simulink model "Boat_Simulation_V1"  (R2015a)
settings: Solver=ode45  StartTime=0.0  StopTime=50  RelTol=1e-3
values from neighbouring files (symbols this model uses):
  d_cg = [0 0 0]    [boatVars.m]
  d_motors = w_boat-0.02    (= 0.06)    [boatVars.m]
  Izz_boat = 1    [boatVars.m]
  k_drag_para = 1    [boatVars.m]
  k_drag_perp = 1    [boatVars.m]
  k_drag_rot = 0.4    [boatVars.m]
  m_boat = 0.120    (= 0.12)    [boatVars.m]
  theta0_boat = 0.*pi/180    (= 0)    [boatVars.m]
  theta_dot0_boat = 0    [boatVars.m]
  use_imu_model = 0    [boatVars.m]
  v0_boat = [0 0]    [boatVars.m]
  x0_boat = waypoints_load(1,:)    [boatVars.m]
  xd = part_pos_2(ii-1,1)    [Baseline_on_Sim.m]    (also in TrackExample.m; TrackExample_revised.m; boatVars.m = 1.5)
  xs = linspace(0,lambda_field,nx)    [boatVars.m]    (also in efficientPath_trials.m = 0:xStep:2*yy; grid_define.m = xmin:step:xmax)
  yd = part_pos_2(ii-1,2)    [Baseline_on_Sim.m]    (also in TrackExample.m; TrackExample_revised.m; boatVars.m = 0.5)
  ys = linspace(0,b_field,ny)    [boatVars.m]    (also in efficientPath_trials.m = 0:yStep:yy; grid_define.m = ymin:step:ymax)
undefined symbols (not defined in the file): b_motor, J_motor, kphi_motor, L_motor, R_motor
libraries: simulink x2, aerolibnav x1
settings Model: Creator=Jack  LastModifiedBy=Jack

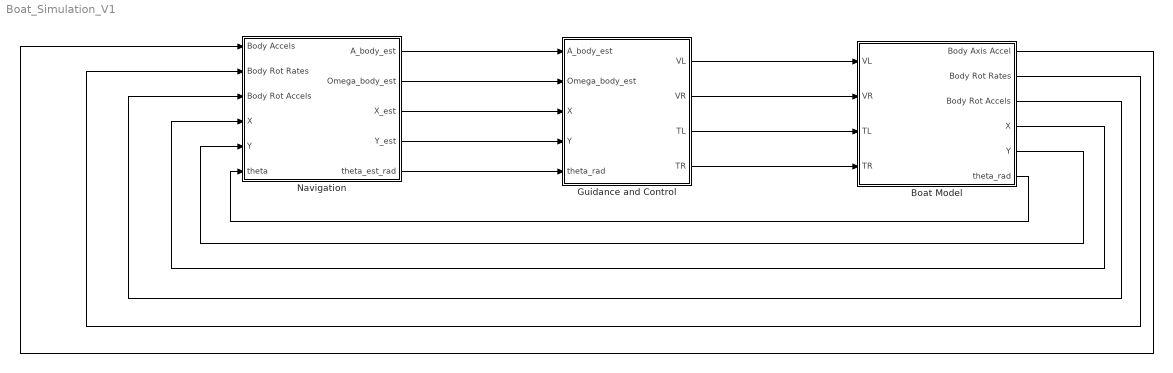
== system Boat_Simulation_V1 ==
  Boat Model : Subsystem
  Guidance and Control : Subsystem
  Navigation : Subsystem
  wires:
  Boat Model/1(Body Axis Accel) -> Navigation/1(Body Accels)
  Boat Model/2(Body Rot Rates) -> Navigation/2(Body Rot Rates)
  Boat Model/3(Body Rot Accels) -> Navigation/3(Body Rot Accels)
  Navigation/1(A_body_est) -> Guidance and Control/1(A_body_est)
  Navigation/2(Omega_body_est) -> Guidance and Control/2(Omega_body_est)
  Guidance and Control/1(VL) -> Boat Model/1(VL)
  Guidance and Control/2(VR) -> Boat Model/2(VR)
  Guidance and Control/3(TL) -> Boat Model/3(TL)
  Guidance and Control/4(TR) -> Boat Model/4(TR)
  Boat Model/4(X) -> Navigation/4(X)
  Boat Model/5(Y) -> Navigation/5(Y)
  Navigation/3(X_est) -> Guidance and Control/3(X)
  Navigation/4(Y_est) -> Guidance and Control/4(Y)
  Navigation/5(theta_est_rad) -> Guidance and Control/5(theta_rad)
  Boat Model/6(theta_rad) -> Navigation/6(theta)

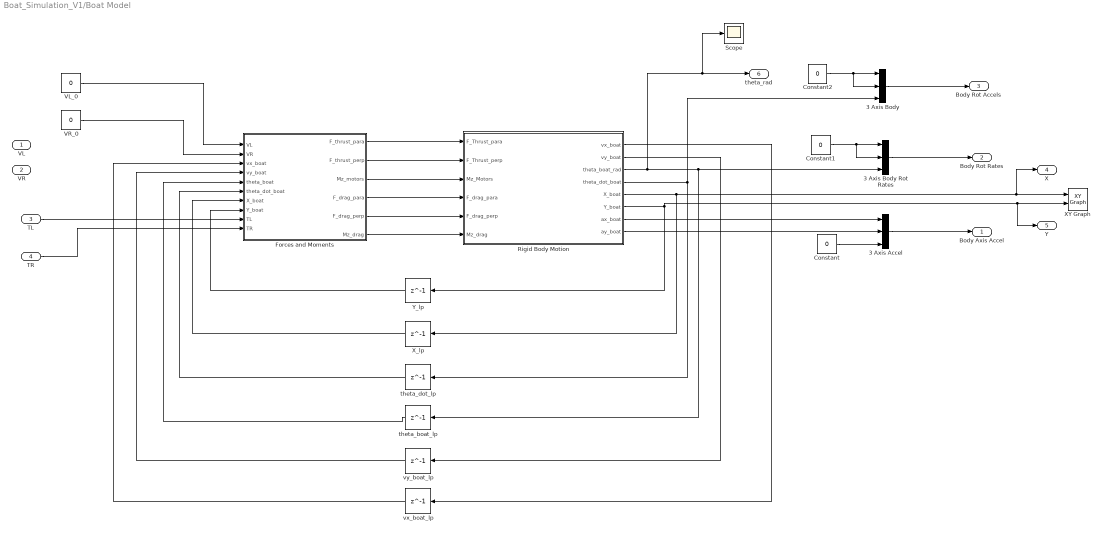
== system Boat_Simulation_V1/Boat Model ==
  VL : Inport
  VR : Inport  Port=2
  TL : Inport  Port=3
  TR : Inport  Port=4
  3 Axis Accel : Concatenate  NumInputs=3
  3 Axis Body : Concatenate  NumInputs=3
  3 Axis Body Rot Rates : Concatenate  NumInputs=3
  Constant : Constant  Value=0
  Constant1 : Constant  Value=0
  Constant2 : Constant  Value=0
  Forces and Moments : Subsystem
  Rigid Body Motion : Subsystem
  Scope : Scope
      settings: SaveName=ScopeData5
  VL_0 : Constant  Value=0
  VR_0 : Constant  Value=0
  XY Graph : simulink/Sinks/XY Graph  xmin=0  xmax=2  ymin=0  ymax=1  st=0.01
  X_lp : Delay  DelayLength=1  InitialCondition=x0_boat(1)  SampleTime=0.01
  Y_lp : Delay  DelayLength=1  InitialCondition=x0_boat(2)  SampleTime=0.01
  theta_boat_lp : Delay  DelayLength=1  InitialCondition=theta0_boat  SampleTime=0.01
  theta_dot_lp : Delay  DelayLength=1  InitialCondition=theta_dot0_boat  SampleTime=0.01
  vx_boat_lp : Delay  DelayLength=1  InitialCondition=v0_boat(1)  SampleTime=0.01
  vy_boat_lp : Delay  DelayLength=1  InitialCondition=v0_boat(2)  SampleTime=0.01
  Body Axis Accel : Outport
  Body Rot Rates : Outport  Port=2
  Body Rot Accels : Outport  Port=3
  X : Outport  Port=4
  Y : Outport  Port=5
  theta_rad : Outport  Port=6
  wires:
  Forces and Moments/3(Mz_motors) -> Rigid Body Motion/3(Mz_Motors)
  Forces and Moments/2(F_thrust_perp) -> Rigid Body Motion/2(F_Thrust_perp)
  Forces and Moments/1(F_thrust_para) -> Rigid Body Motion/1(F_Thrust_para)
  Forces and Moments/4(F_drag_para) -> Rigid Body Motion/4(F_drag_para)
  Forces and Moments/5(F_drag_perp) -> Rigid Body Motion/5(F_drag_perp)
  Forces and Moments/6(Mz_drag) -> Rigid Body Motion/6(Mz_drag)
  Rigid Body Motion/1(vx_boat) -> vx_boat_lp/1
  Rigid Body Motion/2(vy_boat) -> vy_boat_lp/1
  VL_0/1 -> Forces and Moments/1(VL)
  VR_0/1 -> Forces and Moments/2(VR)
  Rigid Body Motion/5(X_boat) -> X_lp/1, X/1, XY Graph/1
  Rigid Body Motion/6(Y_boat) -> Y_lp/1, Y/1, XY Graph/2
  vx_boat_lp/1 -> Forces and Moments/3(vx_boat)
  vy_boat_lp/1 -> Forces and Moments/4(vy_boat)
  theta_boat_lp/1 -> Forces and Moments/5(theta_boat)
  theta_dot_lp/1 -> Forces and Moments/6(theta_dot_boat)
  X_lp/1 -> Forces and Moments/7(X_boat)
  Y_lp/1 -> Forces and Moments/8(Y_boat)
  Rigid Body Motion/7(ax_boat) -> 3 Axis Accel/1
  3 Axis Accel/1 -> Body Axis Accel/1
  Rigid Body Motion/8(ay_boat) -> 3 Axis Accel/2
  Constant/1 -> 3 Axis Accel/3
  3 Axis Body Rot Rates/1 -> Body Rot Rates/1
  Constant1/1 -> 3 Axis Body Rot Rates/2, 3 Axis Body Rot Rates/1
  Rigid Body Motion/4(theta_dot_boat) -> theta_dot_lp/1, 3 Axis Body/3
  3 Axis Body/1 -> Body Rot Accels/1
  Constant2/1 -> 3 Axis Body/2, 3 Axis Body/1
  TL/1 -> Forces and Moments/9(TL)
  TR/1 -> Forces and Moments/10(TR)
  Rigid Body Motion/3(theta_boat_rad) -> Scope/1, theta_rad/1, 3 Axis Body Rot Rates/3, theta_boat_lp/1

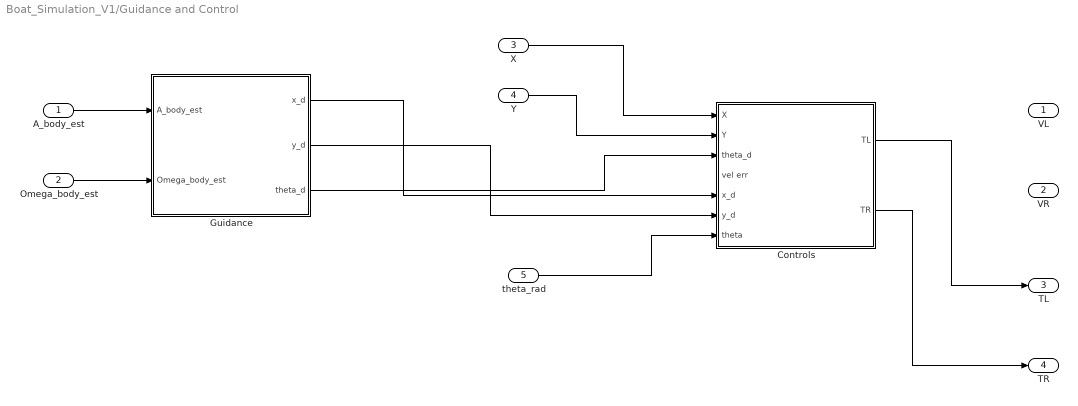
== system Boat_Simulation_V1/Guidance and Control ==
  A_body_est : Inport
  Omega_body_est : Inport  Port=2
  X : Inport  Port=3
  Y : Inport  Port=4
  theta_rad : Inport  Port=5
  Controls : Subsystem
  Guidance : Subsystem
  VL : Outport
  VR : Outport  Port=2
  TL : Outport  Port=3
  TR : Outport  Port=4
  wires:
  Omega_body_est/1 -> Guidance/2("Omega_body_est ")
  A_body_est/1 -> Guidance/1(A_body_est)
  X/1 -> Controls/1(X)
  Y/1 -> Controls/2(Y)
  Guidance/1(x_d) -> Controls/5(x_d)
  Guidance/2(y_d) -> Controls/6(y_d)
  Guidance/3(theta_d) -> Controls/3(theta_d)
  Controls/1(TL) -> TL/1
  Controls/2(TR) -> TR/1
  theta_rad/1 -> Controls/7(theta)

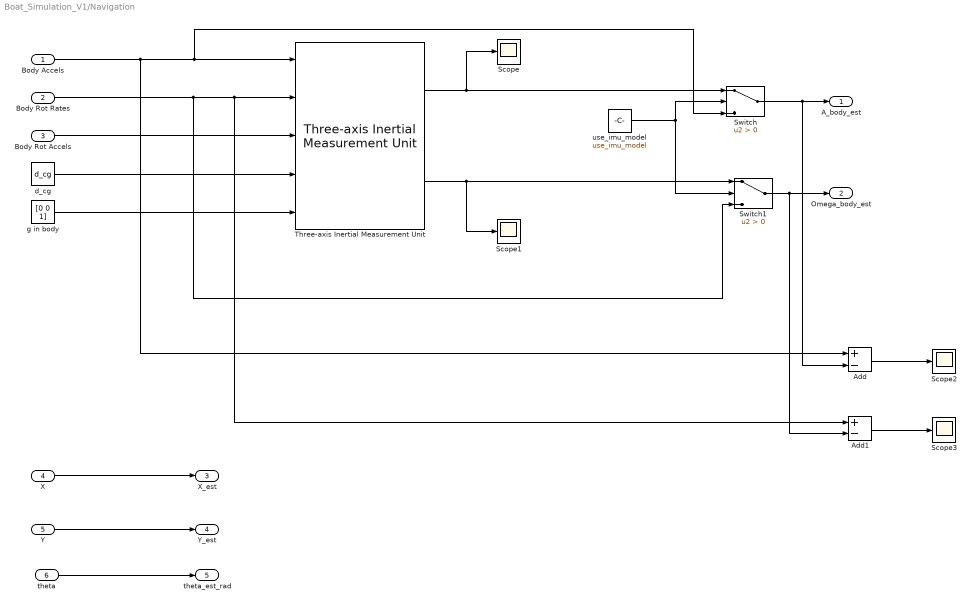
== system Boat_Simulation_V1/Navigation ==
  Body Accels : Inport
  Body Rot Rates : Inport  Port=2
  Body Rot Accels : Inport  Port=3
  X : Inport  Port=4
  Y : Inport  Port=5
  theta : Inport  Port=6
  Add : Sum  Inputs=+-
  Add1 : Sum  Inputs=+-
  Scope{,1..3} (4 alike) : Scope
      Scope settings: ShowLegends=on
      Scope1 settings: ShowLegends=on
      Scope2 settings: SaveName=ScopeData2
      Scope3 settings: SaveName=ScopeData3
  Switch : Switch  Criteria=u2 > Threshold
  Switch1 : Switch  Criteria=u2 > Threshold
  Three-axis Inertial Measurement Unit : aerolibnav/Three-axis Inertial Measurement Unit  units=Metric (MKS)  imu=[0 0 0]  dtype_a=on  w_a=190  z_a=0.707  a_sf_cc=[1 0 0; 0 1 0; 0 0 1]  a_bias=[0 0 0]  a_sat="[-inf  -inf  -inf  inf inf inf]"  dtype_g=on  w_g=190  z_g=0.707  g_sf_cc=[1 0 0; 0 1 0; 0 0 1]  g_bias=[0 0 0]  g_sens=[0 0 0]  g_sat="[-inf  -inf  -inf  inf inf inf]"  i_rand=on  i_seeds=[23093 23094 23095 23096 23097 23098]  i_pow=[0.001 0.001 0.001 0.0001 0.0001 0.0001]  i_Ts=0
  d_cg : Constant  Value=d_cg
  "g in body " : Constant  Value=[0 0 1]
  use_imu_model : Constant  Value=use_imu_model
  A_body_est : Outport
  Omega_body_est : Outport  Port=2
  X_est : Outport  Port=3
  Y_est : Outport  Port=4
  theta_est_rad : Outport  Port=5
  wires:
  Body Accels/1 -> Add/1, Switch/3, Three-axis Inertial Measurement Unit/1
  Body Rot Rates/1 -> Switch1/3, Add1/1, Three-axis Inertial Measurement Unit/2
  Body Rot Accels/1 -> Three-axis Inertial Measurement Unit/3
  "g in body "/1 -> Three-axis Inertial Measurement Unit/5
  d_cg/1 -> Three-axis Inertial Measurement Unit/4
  Three-axis Inertial Measurement Unit/1 -> Switch/1, Scope/1
  Three-axis Inertial Measurement Unit/2 -> Switch1/1, Scope1/1
  Switch1/1 -> Add1/2, Omega_body_est/1
  Switch/1 -> Add/2, A_body_est/1
  use_imu_model/1 -> Switch1/2, Switch/2
  Add/1 -> Scope2/1
  Add1/1 -> Scope3/1
  X/1 -> X_est/1
  Y/1 -> Y_est/1
  theta/1 -> theta_est_rad/1

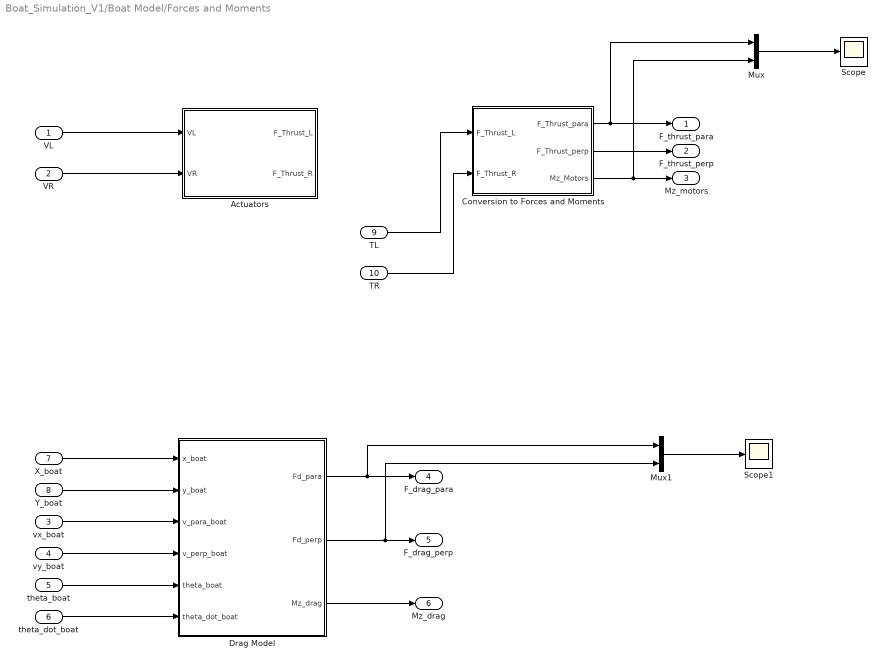
== system Boat_Simulation_V1/Boat Model/Forces and Moments ==
  VL : Inport
  VR : Inport  Port=2
  vx_boat : Inport  Port=3
  vy_boat : Inport  Port=4
  theta_boat : Inport  Port=5
  theta_dot_boat : Inport  Port=6
  X_boat : Inport  Port=7
  Y_boat : Inport  Port=8
  TL : Inport  Port=9
  TR : Inport  Port=10
  Actuators : Subsystem
  Conversion to Forces and Moments : Subsystem
  Drag Model : Subsystem
  Mux : Mux  Inputs=2
  Mux1 : Mux  Inputs=2
  Scope : Scope
      settings: SaveName=ScopeData4
  Scope1 : Scope
      settings: SaveName=ScopeData6
  F_thrust_para : Outport
  F_thrust_perp : Outport  Port=2
  Mz_motors : Outport  Port=3
  F_drag_para : Outport  Port=4
  F_drag_perp : Outport  Port=5
  Mz_drag : Outport  Port=6
  wires:
  VR/1 -> Actuators/2(VR)
  VL/1 -> Actuators/1(VL)
  X_boat/1 -> Drag Model/1(x_boat)
  Y_boat/1 -> Drag Model/2(y_boat)
  vx_boat/1 -> Drag Model/3(v_para_boat)
  vy_boat/1 -> Drag Model/4(v_perp_boat)
  theta_boat/1 -> Drag Model/5(theta_boat)
  Drag Model/3(Mz_drag) -> Mz_drag/1
  Conversion to Forces and Moments/1(F_Thrust_para) -> Mux/1, F_thrust_para/1
  Conversion to Forces and Moments/2(F_Thrust_perp) -> F_thrust_perp/1
  Conversion to Forces and Moments/3(Mz_Motors) -> Mux/2, Mz_motors/1
  theta_dot_boat/1 -> Drag Model/6(theta_dot_boat)
  TL/1 -> Conversion to Forces and Moments/1(F_Thrust_L)
  TR/1 -> Conversion to Forces and Moments/2(F_Thrust_R)
  Mux/1 -> Scope/1
  Drag Model/1(Fd_para) -> Mux1/1, F_drag_para/1
  Drag Model/2(Fd_perp) -> Mux1/2, F_drag_perp/1
  Mux1/1 -> Scope1/1

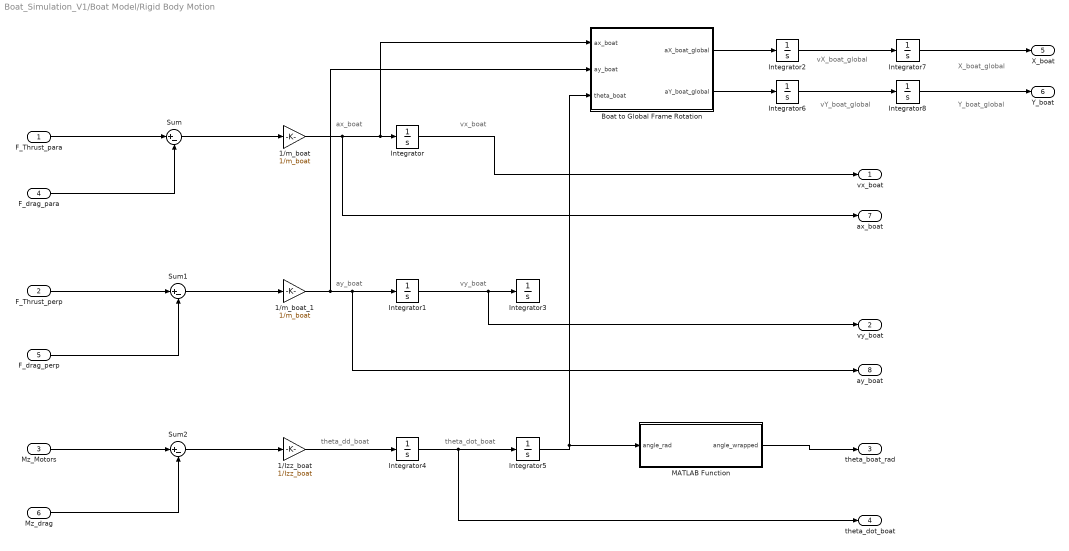
== system Boat_Simulation_V1/Boat Model/Rigid Body Motion ==
  note: Y_boat_global
  note: X_boat_global
  note: vX_boat_global
  note: ax_boat
  note: ay_boat
  note: vx_boat
  note: vy_boat
  note: theta_dd_boat
  note: theta_dot_boat
  note: vY_boat_global
  F_Thrust_para : Inport
  F_Thrust_perp : Inport  Port=2
  Mz_Motors : Inport  Port=3
  F_drag_para : Inport  Port=4
  F_drag_perp : Inport  Port=5
  Mz_drag : Inport  Port=6
  " Boat to Global Frame Rotation" : Subsystem
  1/Izz_boat : Gain  Gain=1/Izz_boat
  1/m_boat : Gain  Gain=1/m_boat
  1/m_boat_1 : Gain  Gain=1/m_boat
  Integrator : Integrator
  Integrator1 : Integrator
  Integrator2 : Integrator  InitialCondition=v0_boat(1)
  Integrator3 : Integrator
  Integrator4 : Integrator  InitialCondition=theta_dot0_boat
  Integrator5 : Integrator  InitialCondition=theta0_boat
  Integrator6 : Integrator  InitialCondition=v0_boat(2)
  Integrator7 : Integrator  InitialCondition=x0_boat(1)  LimitOutput=on  UpperSaturationLimit=2  LowerSaturationLimit=0
  Integrator8 : Integrator  InitialCondition=x0_boat(2)  LimitOutput=on  UpperSaturationLimit=1  LowerSaturationLimit=0
  MATLAB Function : MATLAB Function  TreatAsAtomicUnit=on
  Sum : Sum  Inputs=|+-
  Sum1 : Sum  Inputs=|+-
  Sum2 : Sum  Inputs=|+-
  vx_boat : Outport
  vy_boat : Outport  Port=2
  theta_boat_rad : Outport  Port=3
  theta_dot_boat : Outport  Port=4
  X_boat : Outport  Port=5
  Y_boat : Outport  Port=6
  ax_boat : Outport  Port=7
  ay_boat : Outport  Port=8
  wires:
  F_Thrust_para/1 -> Sum/1
  F_drag_para/1 -> Sum/2
  Sum/1 -> 1/m_boat/1
  Sum1/1 -> 1/m_boat_1/1
  F_Thrust_perp/1 -> Sum1/1
  F_drag_perp/1 -> Sum1/2
  1/m_boat/1 -> ax_boat/1, " Boat to Global Frame Rotation"/1(ax_boat), Integrator/1
  Integrator/1 -> vx_boat/1
  Integrator1/1 -> vy_boat/1, Integrator3/1
  Mz_Motors/1 -> Sum2/1
  Mz_drag/1 -> Sum2/2
  Sum2/1 -> 1/Izz_boat/1
  1/Izz_boat/1 -> Integrator4/1
  Integrator4/1 -> theta_dot_boat/1, Integrator5/1
  Integrator5/1 -> " Boat to Global Frame Rotation"/3(theta_boat), MATLAB Function/1(angle_rad)
  " Boat to Global Frame Rotation"/1(aX_boat_global) -> Integrator2/1
  " Boat to Global Frame Rotation"/2(aY_boat_global) -> Integrator6/1
  Integrator2/1 -> Integrator7/1
  Integrator6/1 -> Integrator8/1
  Integrator7/1 -> X_boat/1
  Integrator8/1 -> Y_boat/1
  1/m_boat_1/1 -> " Boat to Global Frame Rotation"/2(ay_boat), ay_boat/1, Integrator1/1
  MATLAB Function/1(angle_wrapped) -> theta_boat_rad/1

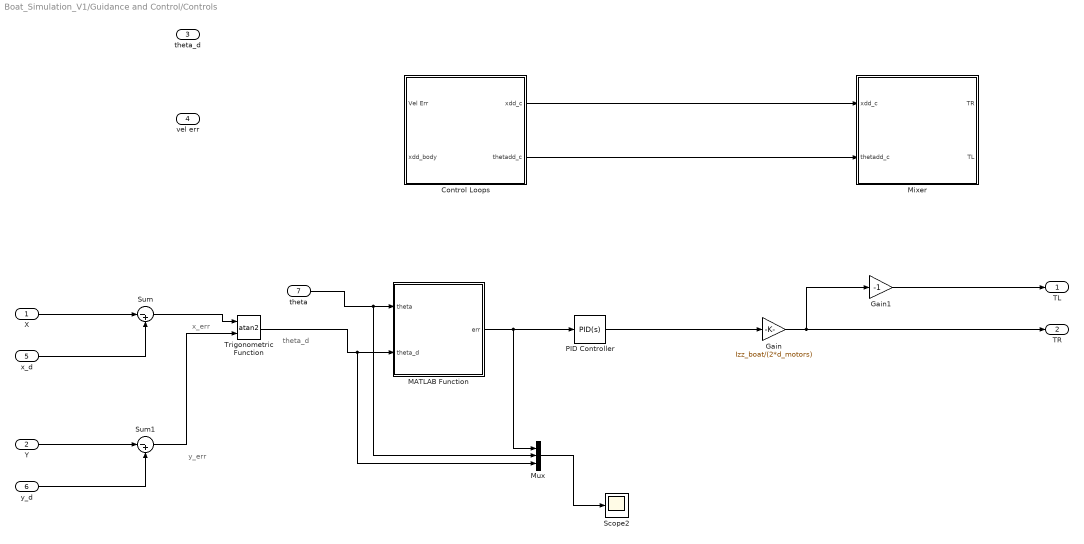
== system Boat_Simulation_V1/Guidance and Control/Controls ==
  note: theta_d
  note: y_err
  note: x_err
  X : Inport
  Y : Inport  Port=2
  theta_d : Inport  Port=3
  vel err : Inport  Port=4
  x_d : Inport  Port=5
  y_d : Inport  Port=6
  theta : Inport  Port=7
  Control Loops : Subsystem
  Gain : Gain  Gain=Izz_boat/(2*d_motors)
  Gain1 : Gain  Gain=-1
  MATLAB Function : MATLAB Function  TreatAsAtomicUnit=on
  Mixer : Subsystem
  Mux : Mux  Inputs=3
  PID Controller : simulink/Continuous/PID Controller  Controller=PID  TimeDomain=Continuous-time  SampleTime=-1  IntegratorMethod=Forward Euler  FilterMethod=Forward Euler  Form=Parallel  UseFilter=on  ControllerParametersSource=internal  P=0.3  I=0.1  D=0  N=100  InitialConditionSource=internal  InitialConditionForIntegrator=0  InitialConditionForFilter=0  ExternalReset=none  LimitOutput=off  UpperSaturationLimit=inf  LowerSaturationLimit=-inf  LinearizeAsGain=on  AntiWindupMode=none  Kb=1  TrackingMode=off  Kt=1  PParamMin=[]  PParamMax=[]  IParamMin=[]  IParamMax=[]  DParamMin=[]  DParamMax=[]  NParamMin=[]  NParamMax=[]  KbParamMin=[]  KbParamMax=[]  KtParamMin=[]  KtParamMax=[]  POutMin=[]  POutMax=[]  IOutMin=[]  IOutMax=[]  DOutMin=[]  DOutMax=[]  NOutMin=[]  NOutMax=[]  KbOutMin=[]  KbOutMax=[]  KtOutMin=[]  KtOutMax=[]  IntegratorOutMin=[]  IntegratorOutMax=[]  FilterOutMin=[]  FilterOutMax=[]  SumOutMin=[]  SumOutMax=[]  SumI1OutMin=[]  SumI1OutMax=[]  SumI2OutMin=[]  SumI2OutMax=[]  SumI3OutMin=[]  SumI3OutMax=[]  SumDOutMin=[]  SumDOutMax=[]  SaturationOutMin=[]  SaturationOutMax=[]  IntegratorContinuousStateAttributes=''  IntegratorStateMustResolveToSignalObject=off  IntegratorRTWStateStorageClass=Auto  FilterContinuousStateAttributes=''  FilterStateMustResolveToSignalObject=off  FilterRTWStateStorageClass=Auto  DifferentiatorICPrevScaledInput=0  DifferentiatorOutMin=[]  DifferentiatorOutMax=[]
  Scope2 : Scope
      settings: ShowLegends=on  SaveName=ScopeData9
  Sum : Sum  Inputs=|-+
  Sum1 : Sum  Inputs=|-+
  Trigonometric Function : Trigonometry  Operator=atan2
  TL : Outport
  TR : Outport  Port=2
  wires:
  Control Loops/1(xdd_c) -> Mixer/1(xdd_c)
  Control Loops/2(thetadd_c) -> Mixer/2(thetadd_c)
  X/1 -> Sum/1
  x_d/1 -> Sum/2
  Y/1 -> Sum1/1
  y_d/1 -> Sum1/2
  PID Controller/1 -> Gain/1
  Gain/1 -> TR/1, Gain1/1
  theta/1 -> Mux/2, MATLAB Function/1(theta)
  Sum/1 -> Trigonometric Function/1
  Sum1/1 -> Trigonometric Function/2
  Gain1/1 -> TL/1
  Mux/1 -> Scope2/1
  MATLAB Function/1(err) -> Mux/1, PID Controller/1
  Trigonometric Function/1 -> Mux/3, MATLAB Function/2(theta_d)

== system Boat_Simulation_V1/Guidance and Control/Guidance ==
  A_body_est : Inport
  "Omega_body_est " : Inport  Port=2
  Sine Wave : Sin  Amplitude=pi  Frequency=2*pi/50  SampleTime=0
  xd : Constant  Value=xd
  yd : Constant  Value=yd
  x_d : Outport
  y_d : Outport  Port=2
  theta_d : Outport  Port=3
  wires:
  xd/1 -> x_d/1
  yd/1 -> y_d/1
  Sine Wave/1 -> theta_d/1

== system Boat_Simulation_V1/Boat Model/Forces and Moments/Actuators ==
  note: Left Motor
  note: Right Motor
  VL : Inport
  VR : Inport  Port=2
  DC motor : Subsystem  mask(DC Motor){L=L_motor, Kphi=kphi_motor, J=J_motor, b=b_motor, R=R_motor}
      mask help:
      | Takes the DC voltage as input, and outputs angular velocity (w) and current (i)
      | L => windings inductance		Kphi => emf constant
      | J => loads moment of inertial		b => viscous friction
      | R => windings resistance
      mask Display:
      | port_label('input', 1, 'V')
      | port_label('output', 2, 'i')
      | port_label('output', 1, 'w')
      | disp('DC Motor')
  DC motor1 : Subsystem  mask(DC Motor){L=L_motor, Kphi=kphi_motor, J=J_motor, b=b_motor, R=R_motor}
      mask help:
      | Takes the DC voltage as input, and outputs angular velocity (w) and current (i)
      | L => windings inductance		Kphi => emf constant
      | J => loads moment of inertial		b => viscous friction
      | R => windings resistance
      mask Display:
      | port_label('input', 1, 'V')
      | port_label('output', 2, 'i')
      | port_label('output', 1, 'w')
      | disp('DC Motor')
  Prop Angular Velocity to Thrust : Lookup_n-D  NumberOfTableDimensions=1  BreakpointsForDimension1=[-5:5]  Table=tanh([-5:5])  InternalRulePriority=Speed  RndMeth=Simplest  InputSameDT=on
  Prop Angular Velocity to Thrust1 : Lookup_n-D  NumberOfTableDimensions=1  BreakpointsForDimension1=[-5:5]  Table=tanh([-5:5])  InternalRulePriority=Speed  RndMeth=Simplest  InputSameDT=on
  F_Thrust_L : Outport
  F_Thrust_R : Outport  Port=2
  wires:
  DC motor/1(w) -> Prop Angular Velocity to Thrust/1
  DC motor1/1(w) -> Prop Angular Velocity to Thrust1/1
  VL/1 -> DC motor/1(V)
  VR/1 -> DC motor1/1(V)
  Prop Angular Velocity to Thrust/1 -> F_Thrust_L/1
  Prop Angular Velocity to Thrust1/1 -> F_Thrust_R/1

== system Boat_Simulation_V1/Boat Model/Forces and Moments/Conversion to Forces and Moments ==
  F_Thrust_L : Inport
  F_Thrust_R : Inport  Port=2
  Constant : Constant  Value=0
  Divide : Product  Inputs=*/
  Sum : Sum  Inputs=|++
  Sum1 : Sum  Inputs=+-|
  d_motors/2 : Constant  Value=d_motors/2
  F_Thrust_para : Outport
  F_Thrust_perp : Outport  Port=2
  Mz_Motors : Outport  Port=3
  wires:
  F_Thrust_L/1 -> Sum1/1, Sum/1
  F_Thrust_R/1 -> Sum1/2, Sum/2
  Sum/1 -> F_Thrust_para/1
  Constant/1 -> F_Thrust_perp/1
  Sum1/1 -> Divide/1
  d_motors/2/1 -> Divide/2
  Divide/1 -> Mz_Motors/1

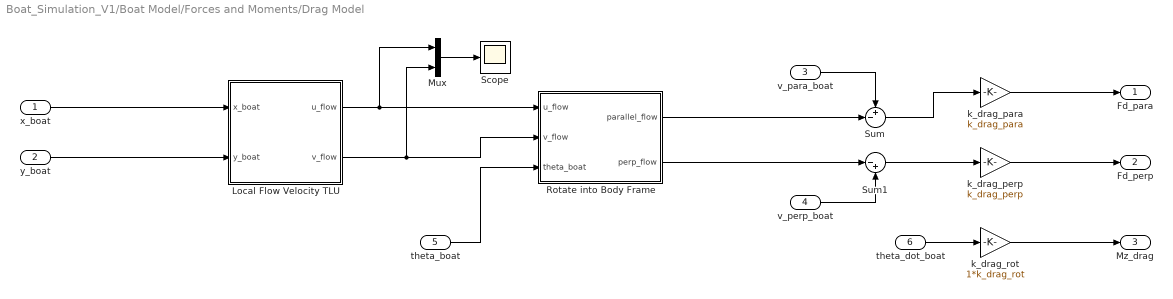
== system Boat_Simulation_V1/Boat Model/Forces and Moments/Drag Model ==
  x_boat : Inport
  y_boat : Inport  Port=2
  v_para_boat : Inport  Port=3
  v_perp_boat : Inport  Port=4
  theta_boat : Inport  Port=5
  theta_dot_boat : Inport  Port=6
  Local Flow Velocity TLU : Subsystem
  Mux : Mux  Inputs=2
  "Rotate into Body Frame " : Subsystem
  Scope : Scope
      settings: SaveName=ScopeData7
  Sum : Sum  Inputs=+-|
  Sum1 : Sum  Inputs=|-+
  k_drag_para : Gain  Gain=k_drag_para
  k_drag_perp : Gain  Gain=k_drag_perp
  k_drag_rot : Gain  Gain=1*k_drag_rot
  Fd_para : Outport
  Fd_perp : Outport  Port=2
  Mz_drag : Outport  Port=3
  wires:
  x_boat/1 -> Local Flow Velocity TLU/1(x_boat)
  y_boat/1 -> Local Flow Velocity TLU/2(y_boat)
  Sum/1 -> k_drag_para/1
  Sum1/1 -> k_drag_perp/1
  Local Flow Velocity TLU/1(u_flow) -> Mux/1, "Rotate into Body Frame "/1(u_flow)
  Local Flow Velocity TLU/2(v_flow) -> Mux/2, "Rotate into Body Frame "/2(v_flow)
  theta_boat/1 -> "Rotate into Body Frame "/3(theta_boat)
  "Rotate into Body Frame "/1(parallel_flow) -> Sum/2
  "Rotate into Body Frame "/2(perp_flow) -> Sum1/1
  theta_dot_boat/1 -> k_drag_rot/1
  k_drag_rot/1 -> Mz_drag/1
  k_drag_para/1 -> Fd_para/1
  k_drag_perp/1 -> Fd_perp/1
  v_para_boat/1 -> Sum/1
  v_perp_boat/1 -> Sum1/2
  Mux/1 -> Scope/1

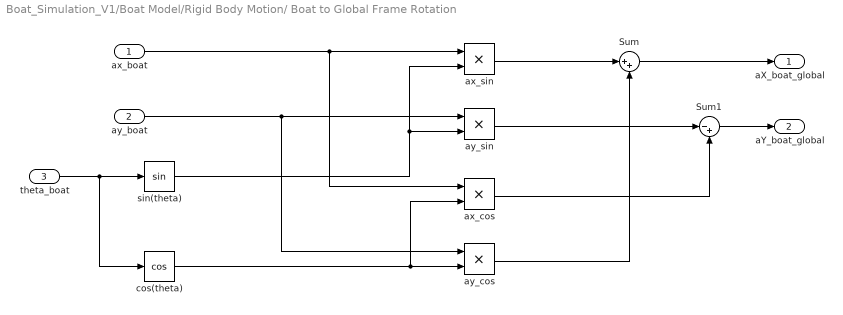
== system Boat_Simulation_V1/Boat Model/Rigid Body Motion/ Boat to Global Frame Rotation ==
  ax_boat : Inport
  ay_boat : Inport  Port=2
  theta_boat : Inport  Port=3
  Sum : Sum  Inputs=|++
  Sum1 : Sum  Inputs=|-+
  ax_cos : Product
  ax_sin : Product
  ay_cos : Product
  ay_sin : Product
  cos(theta) : Trigonometry  Operator=cos  ApproximationMethod=CORDIC
  sin(theta) : Trigonometry  ApproximationMethod=CORDIC
  aX_boat_global : Outport
  aY_boat_global : Outport  Port=2
  wires:
  theta_boat/1 -> cos(theta)/1, sin(theta)/1
  ax_boat/1 -> ax_cos/1, ax_sin/1
  sin(theta)/1 -> ax_sin/2, ay_sin/2
  cos(theta)/1 -> ay_cos/2, ax_cos/2
  ay_boat/1 -> ay_cos/1, ay_sin/1
  Sum/1 -> aX_boat_global/1
  Sum1/1 -> aY_boat_global/1
  ax_sin/1 -> Sum/1
  ay_cos/1 -> Sum/2
  ax_cos/1 -> Sum1/2
  ay_sin/1 -> Sum1/1

== system Boat_Simulation_V1/Guidance and Control/Controls/Control Loops ==
  Vel Err : Inport
  xdd_body : Inport  Port=2
  Axial Velocity Loop : Subsystem
  Rotation Loop : Subsystem
  xdd_c : Outport
  thetadd_c : Outport  Port=2
  wires:
  Rotation Loop/1(thetadd_c) -> thetadd_c/1
  Axial Velocity Loop/1(vdot_c) -> xdd_c/1
  Vel Err/1 -> Axial Velocity Loop/1(Vel Err)
  xdd_body/1 -> Axial Velocity Loop/2(vdot_body)

== system Boat_Simulation_V1/Guidance and Control/Controls/Mixer ==
  xdd_c : Inport
  thetadd_c : Inport  Port=2
  TR : Outport
  TL : Outport  Port=2

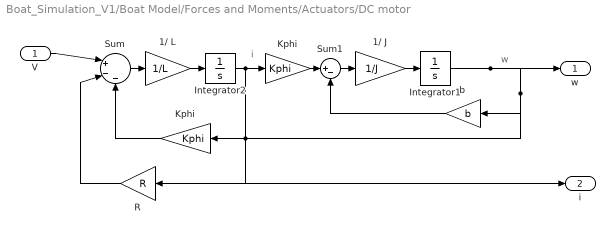
== system Boat_Simulation_V1/Boat Model/Forces and Moments/Actuators/DC motor ==
  note: i
  note: w
  V : Inport
  1/ J : Gain  Gain=1/J
  1/ L : Gain  Gain=1/L
  Integrator1 : Integrator
  Integrator2 : Integrator
  Kphi : Gain  Gain=Kphi
  "Kphi " : Gain  Gain=Kphi
  R : Gain  Gain=R
  Sum : Sum  Inputs=|+--
  Sum1 : Sum  Inputs=|+-
  b : Gain  Gain=b
  w : Outport
  i : Outport  Port=2
  wires:
  V/1 -> Sum/1
  Sum/1 -> 1/ L/1
  1/ L/1 -> Integrator2/1
  Integrator2/1 -> Kphi/1, R/1, i/1
  Kphi/1 -> Sum1/1
  Sum1/1 -> 1/ J/1
  1/ J/1 -> Integrator1/1
  Integrator1/1 -> "Kphi "/1, b/1, w/1
  b/1 -> Sum1/2
  "Kphi "/1 -> Sum/3
  R/1 -> Sum/2

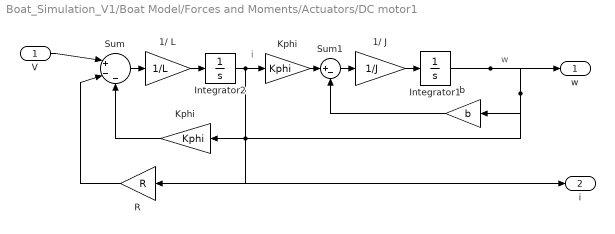
== system Boat_Simulation_V1/Boat Model/Forces and Moments/Actuators/DC motor1 ==
  note: i
  note: w
  V : Inport
  1/ J : Gain  Gain=1/J
  1/ L : Gain  Gain=1/L
  Integrator1 : Integrator
  Integrator2 : Integrator
  Kphi : Gain  Gain=Kphi
  "Kphi " : Gain  Gain=Kphi
  R : Gain  Gain=R
  Sum : Sum  Inputs=|+--
  Sum1 : Sum  Inputs=|+-
  b : Gain  Gain=b
  w : Outport
  i : Outport  Port=2
  wires:
  V/1 -> Sum/1
  Sum/1 -> 1/ L/1
  1/ L/1 -> Integrator2/1
  Integrator2/1 -> Kphi/1, R/1, i/1
  Kphi/1 -> Sum1/1
  Sum1/1 -> 1/ J/1
  1/ J/1 -> Integrator1/1
  Integrator1/1 -> "Kphi "/1, b/1, w/1
  b/1 -> Sum1/2
  "Kphi "/1 -> Sum/3
  R/1 -> Sum/2

== system Boat_Simulation_V1/Boat Model/Forces and Moments/Drag Model/Local Flow Velocity TLU ==
  x_boat : Inport
  y_boat : Inport  Port=2
  U_field : Lookup_n-D  BreakpointsForDimension1=xs  BreakpointsForDimension2=ys  BeginIndexSearchUsingPreviousIndexResult=on  Table=U_field'  ExtrapMethod=Clip  UseLastTableValue=on  InternalRulePriority=Speed  RndMeth=Simplest  InputSameDT=on
  V_field : Lookup_n-D  BreakpointsForDimension1=xs  BreakpointsForDimension2=ys  BeginIndexSearchUsingPreviousIndexResult=on  Table=V_field_load'  ExtrapMethod=Clip  UseLastTableValue=on  InternalRulePriority=Speed  RndMeth=Simplest  InputSameDT=on
  u_flow : Outport
  v_flow : Outport  Port=2
  wires:
  U_field/1 -> u_flow/1
  V_field/1 -> v_flow/1
  x_boat/1 -> U_field/1, V_field/1
  y_boat/1 -> V_field/2, U_field/2

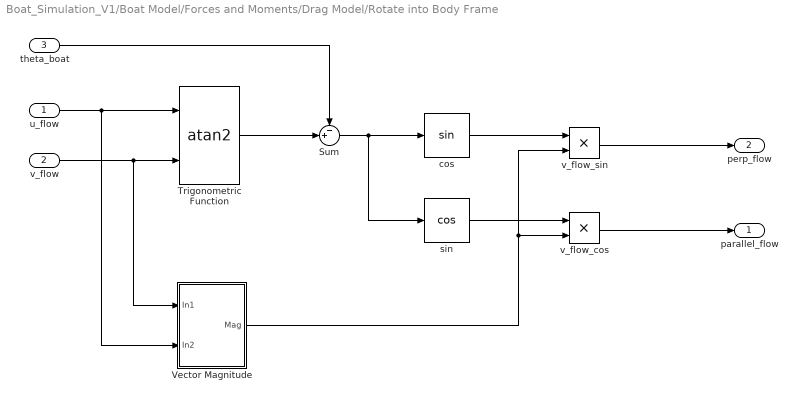
== system Boat_Simulation_V1/Boat Model/Forces and Moments/Drag Model/Rotate into Body Frame  ==
  u_flow : Inport
  v_flow : Inport  Port=2
  theta_boat : Inport  Port=3
  Sum : Sum  Inputs=-+|
  Trigonometric Function : Trigonometry  Operator=atan2
  Vector Magnitude : Subsystem
  "cos " : Trigonometry
  sin : Trigonometry  Operator=cos
  v_flow_cos : Product  Inputs=**
  v_flow_sin : Product  Inputs=**
  parallel_flow : Outport
  perp_flow : Outport  Port=2
  wires:
  v_flow/1 -> Vector Magnitude/1(In1), Trigonometric Function/2
  u_flow/1 -> Trigonometric Function/1, Vector Magnitude/2(In2)
  Trigonometric Function/1 -> Sum/2
  theta_boat/1 -> Sum/1
  Sum/1 -> sin/1, "cos "/1
  "cos "/1 -> v_flow_sin/1
  sin/1 -> v_flow_cos/1
  Vector Magnitude/1(Mag) -> v_flow_sin/2, v_flow_cos/2
  v_flow_sin/1 -> perp_flow/1
  v_flow_cos/1 -> parallel_flow/1

== system Boat_Simulation_V1/Guidance and Control/Controls/Control Loops/Axial Velocity Loop ==
  Vel Err : Inport
  vdot_body : Inport  Port=2
  Deaug : Subsystem
  vdot_c : Outport

== system Boat_Simulation_V1/Guidance and Control/Controls/Control Loops/Rotation Loop ==
  In1 : Inport
  thetadd_c : Outport
  wires:
  In1/1 -> thetadd_c/1

== system Boat_Simulation_V1/Boat Model/Forces and Moments/Drag Model/Rotate into Body Frame /Vector Magnitude ==
  In1 : Inport
  In2 : Inport  Port=2
  Math Function : Math  Operator=square  SaturateOnIntegerOverflow=on
  Math Function1 : Math  Operator=square  SaturateOnIntegerOverflow=on
  Sqrt : Sqrt  SaturateOnIntegerOverflow=on
  Sum1 : Sum
  Mag : Outport
  wires:
  Math Function/1 -> Sum1/1
  In1/1 -> Math Function/1
  Sqrt/1 -> Mag/1
  In2/1 -> Math Function1/1
  Math Function1/1 -> Sum1/2
  Sum1/1 -> Sqrt/1

== system Boat_Simulation_V1/Guidance and Control/Controls/Control Loops/Axial Velocity Loop/Deaug ==
  In1 : Inport
  Out1 : Outport
  wires:
  In1/1 -> Out1/1

== matlab function Boat_Simulation_V1/Boat Model/Rigid Body Motion/MATLAB Function ==
  data: angle_rad input; angle_wrapped output
function angle_wrapped = wrap2pi(angle_rad)
    angle_wrapped = angle_rad - 2*pi*floor( (angle_rad+pi)/(2*pi) ); 
end

== matlab function Boat_Simulation_V1/Guidance and Control/Controls/MATLAB Function ==
  data: theta input; err output; theta_d input
function err = turnCorrection(theta,theta_d)
    if (theta>0 && theta_d<0 && abs(theta-theta_d)>pi)
        err = -(2*pi-abs(theta-theta_d));
    elseif (theta<0 && theta_d>0 && abs(theta-theta_d)>pi)
        err = (2*pi-abs(theta-theta_d));
    else
        err = theta-theta_d;
    end
end
